simulink model "homework"  (R2019b)
settings: Solver=VariableStepAuto  StartTime=0.0  StopTime=10.0  RelTol=1e-3
values from neighbouring files (symbols this model uses):
  b = 0.5e-3    (= 0.0005)    [Untitled.m]
  i = 0.022    [Untitled.m]
  kb = 1.2    [Untitled.m]
  kt = 1.2    [Untitled.m]
  l = 0.035    [Untitled.m]
  r = 2.45    [Untitled.m]
settings Model: Creator=ASUS  LastModifiedBy=ASUS

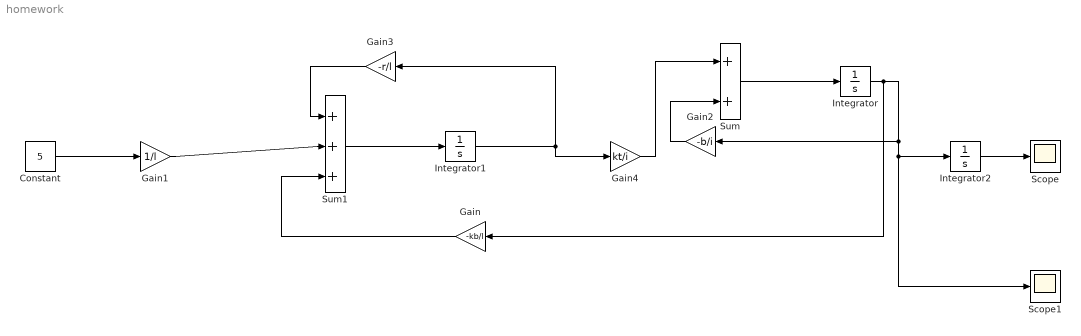
== system homework ==
  Constant : Constant  Value=5
  Gain : Gain  Gain=-kb/l
  Gain1 : Gain  Gain=1/l
  Gain2 : Gain  Gain=-b/i
  Gain3 : Gain  Gain=-r/l
  Gain4 : Gain  Gain=kt/i
  Integrator : Integrator
  Integrator1 : Integrator
  Integrator2 : Integrator
  Scope : Scope
  Scope1 : Scope
  Sum : Sum  Inputs=|++
  Sum1 : Sum  Inputs=|+++
  wires:
  Constant/1 -> Gain1/1
  Gain1/1 -> Sum1/2
  Sum1/1 -> Integrator1/1
  Integrator1/1 -> Gain4/1, Gain3/1
  Sum/1 -> Integrator/1
  Integrator/1 -> Gain/1, Gain2/1, Scope1/1, Integrator2/1
  Gain2/1 -> Sum/2
  Gain/1 -> Sum1/3
  Gain3/1 -> Sum1/1
  Gain4/1 -> Sum/1
  Integrator2/1 -> Scope/1
